simulink model "ThesisControlModel"  (R2024b)
settings: Solver=VariableStepAuto  StartTime=0.0  StopTime=100  RelTol=1e-3
model workspace (MAT data in the model file):
  Ts = 0.15
  k = 0.035
  ki = 0.01
settings Model: Creator=flyingtopher  LastModifiedBy=flyingtopher

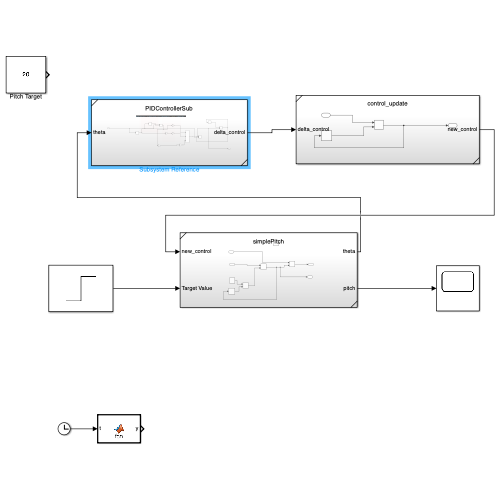
[thumbnail: Simulink's stored preview of the top-level diagram]
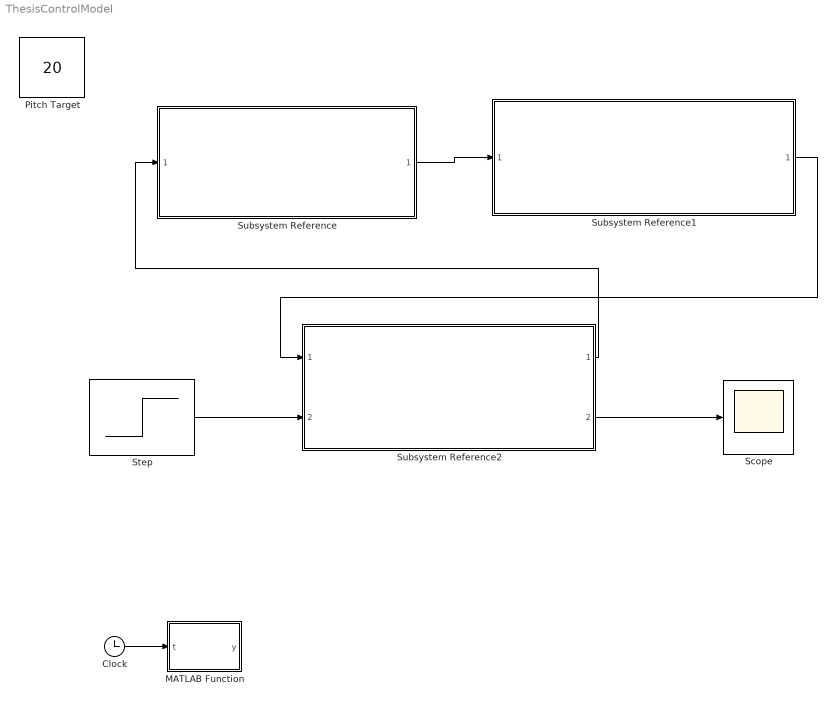
== system ThesisControlModel ==
  Clock : Clock
  MATLAB Function : MATLAB Function  TreatAsAtomicUnit=on
  Pitch Target : Constant  Value=20
  Scope : Scope
  Step : Step  Time=25  Before=10  After=25  SampleTime=0
  Subsystem Reference : Subsystem  ReferencedSubsystem=PIDControllerSub
  Subsystem Reference1 : Subsystem  ReferencedSubsystem=control_update
  Subsystem Reference2 : Subsystem  ReferencedSubsystem=simplePitch
  wires:
  Subsystem Reference/1 -> Subsystem Reference1/1
  Subsystem Reference1/1 -> Subsystem Reference2/1
  Subsystem Reference2/1 -> Subsystem Reference/1
  Subsystem Reference2/2 -> Scope/1
  Clock/1 -> MATLAB Function/1(t)
  Step/1 -> Subsystem Reference2/2

== matlab function ThesisControlModel/MATLAB Function ==
  data: t input; y output
function y = fcn(t)
a = 20;
b = 10;
c = 3;
t = t - a;
y = 0;
if t > 0
    y = ceil(t/c)*b;
end
